simulink model "fdm"  (R2020b)
settings: Solver=VariableStepAuto  StartTime=0.0  StopTime=3  RelTol=1e-3
InitFcn:
  | clear all
  | close all
  | clc
  | fs=44100;
  | ts=1/fs;
libraries: dsparch4 x10, dspvision x4, commchan3 x1
settings Model: Creator=tamim  LastModifiedBy=Safir
settings DebuggingCC: SFMachineParentedDataDiag=error

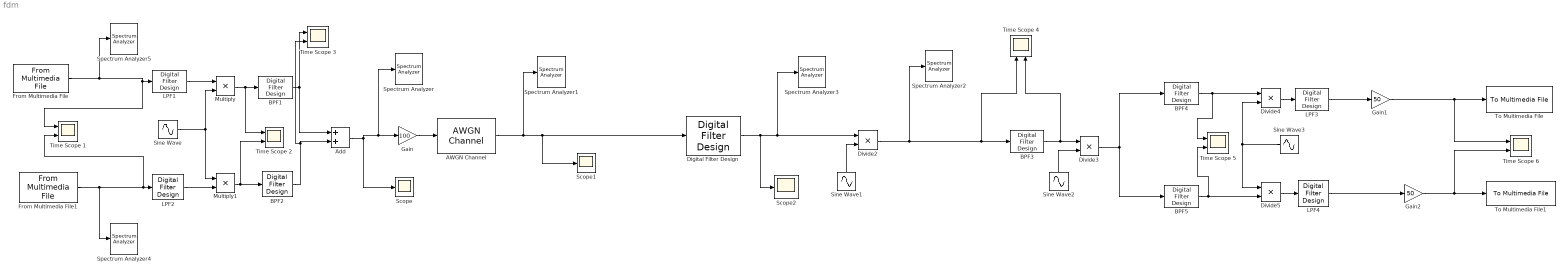
== system fdm ==
  AWGN Channel : commchan3/AWGN Channel  InputProcessing=Columns as channels (frame based)  seed=67  noiseMode="Signal to noise ratio  (SNR)"  EbNodB=10  EsNodB=10  SNRdB=-3  bitsPerSym=1  Ps=1  Tsym=1  variance=1
  Add : Sum  SampleTime=ts
  BPF{1..5} (5 alike) : dsparch4/Digital Filter Design  mwdsp_browser_bugfix_var=off
  Digital Filter Design : dsparch4/Digital Filter Design  mwdsp_browser_bugfix_var=off
  Divide{2..5} (4 alike) : Product  Inputs=**  SampleTime=ts
  From Multimedia File : dspvision/From Multimedia File  inputFilename=C:\Users\Safir\Desktop\L-3,T-1\EEE 310 COMMUNICATION LAB\Project\Our works\Project Codes\test.wav  readRange=[1 Inf]  loop=on  numPlays=inf  outputStreams=Audio only  videoDataType=single  audioDataType=double  inheritSampleTime=on  userDefinedSampleTime=1/30  noAudioOutput=off  isIntensityVideo=off  fourcc=RGB  colorVideoFormat=Separate color signals  outputEOF=off  dataOrg=Column-major  audioFrameSize=1  computeAudioFrameSize=off  outSamplingMode=Sample based
  From Multimedia File1 : dspvision/From Multimedia File  inputFilename=C:\Users\Safir\Desktop\L-3,T-1\EEE 310 COMMUNICATION LAB\Project\Our works\Project Codes\speech_dft.wav  readRange=[1 Inf]  loop=on  numPlays=inf  outputStreams=Audio only  videoDataType=single  audioDataType=double  inheritSampleTime=on  userDefinedSampleTime=1/30  noAudioOutput=off  isIntensityVideo=off  fourcc=RGB  colorVideoFormat=Separate color signals  outputEOF=off  dataOrg=Column-major  audioFrameSize=1  computeAudioFrameSize=off  outSamplingMode=Sample based
  Gain : Gain  Gain=100
  Gain1 : Gain  Gain=50
  Gain2 : Gain  Gain=50
  LPF{1..4} (4 alike) : dsparch4/Digital Filter Design  mwdsp_browser_bugfix_var=off
  Multiply : Product  Inputs=**  SampleTime=ts
  Multiply1 : Product  Inputs=**  SampleTime=ts
  Scope : Scope
  Scope1 : Scope
  Scope2 : Scope
  Sine Wave : Sin  Frequency=2*pi*6000  SampleTime=ts
  Sine Wave1 : Sin  Frequency=2*pi*12000  SampleTime=ts
  Sine Wave2 : Sin  Frequency=2*pi*12000  SampleTime=ts
  Sine Wave3 : Sin  Frequency=2*pi*6000  SampleTime=ts
  Spectrum Analyzer{,1..5} (6 alike) : SpectrumAnalyzer
  Time Scope {1..6} (6 alike) : Scope  NumInputPorts=2
  To Multimedia File : dspvision/To Multimedia File  outputFilename=C:\Users\Safir\Desktop\L-3,T-1\EEE 310 COMMUNICATION LAB\Project\Our works\Project Codes\recons1.wav  streamSelection=Audio only  videoCompressor=None (uncompressed)  audioCompressor=None (uncompressed)  imagePorts=One multidimensional signal  fileType=WAV  audioDatatype=16-bit integer  fourcc=RGB  videoQuality=75  mj2000CompFactor=10
  To Multimedia File1 : dspvision/To Multimedia File  outputFilename=C:\Users\Safir\Desktop\L-3,T-1\EEE 310 COMMUNICATION LAB\Project\Our works\Project Codes\recons2.wav  streamSelection=Audio only  videoCompressor=Lossy  audioCompressor=None (uncompressed)  imagePorts=One multidimensional signal  fileType=WAV  audioDatatype=16-bit integer  fourcc=RGB  videoQuality=75  mj2000CompFactor=10
  wires:
  BPF2/1 -> Add/2, Time Scope 3/2
  BPF1/1 -> Time Scope 3/1, Add/1
  From Multimedia File/1 -> Spectrum Analyzer5/1, Time Scope 1/1, LPF1/1
  Sine Wave/1 -> Multiply1/1, Multiply/2
  Sine Wave1/1 -> Divide2/2
  LPF4/1 -> Gain2/1
  Divide2/1 -> Spectrum Analyzer2/1, Time Scope 4/1, BPF3/1
  Sine Wave3/1 -> Divide5/1, Divide4/2
  Divide5/1 -> LPF4/1
  BPF4/1 -> Time Scope 5/1, Divide4/1
  BPF3/1 -> Divide3/1, Time Scope 4/2
  Divide4/1 -> LPF3/1
  Multiply1/1 -> Time Scope 2/2, BPF2/1
  Multiply/1 -> Time Scope 2/1, BPF1/1
  BPF5/1 -> Time Scope 5/2, Divide5/2
  Divide3/1 -> BPF5/1, BPF4/1
  LPF1/1 -> Multiply/1
  Sine Wave2/1 -> Divide3/2
  LPF2/1 -> Multiply1/2
  From Multimedia File1/1 -> Spectrum Analyzer4/1, Time Scope 1/2, LPF2/1
  LPF3/1 -> Gain1/1
  Add/1 -> Spectrum Analyzer/1, Gain/1, Scope/1
  AWGN Channel/1 -> Spectrum Analyzer1/1, Scope1/1, Digital Filter Design/1
  Digital Filter Design/1 -> Scope2/1, Spectrum Analyzer3/1, Divide2/1
  Gain/1 -> AWGN Channel/1
  Gain2/1 -> Time Scope 6/2, To Multimedia File1/1
  Gain1/1 -> Time Scope 6/1, To Multimedia File/1
